simulink model "LQR"  (R2023a)
settings: Solver=ode23t  StartTime=0.0  StopTime=1.1  MaxStep=0.1  RelTol=1e-4
undefined symbols (not defined in the file): LQR_parameters, State_space
settings Model: Creator=ПК  LastModifiedBy=ПК

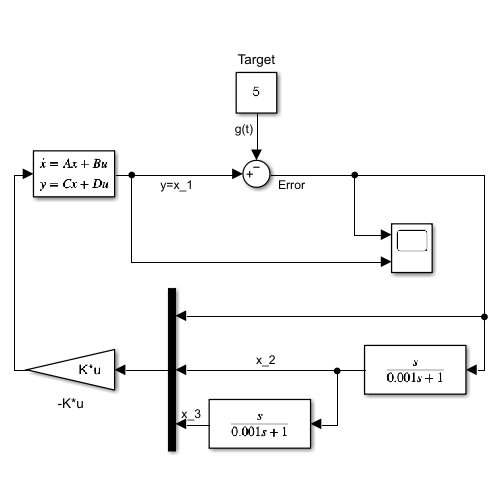
[thumbnail: Simulink's stored preview of the top-level diagram]
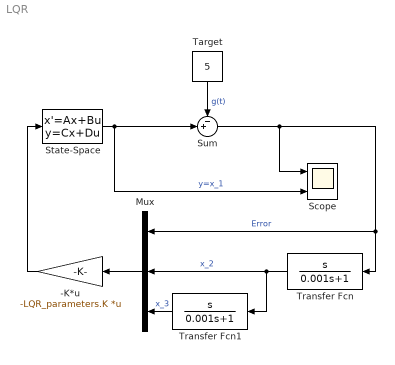
== system LQR ==
  -K*u : Gain  Gain=-LQR_parameters.K  Multiplication=Matrix(K*u)
  Mux : Mux  Inputs=3
  Scope : Scope  NumInputPorts=2
  State-Space : StateSpace  A=State_space.A  B=State_space.B  C=State_space.C  D=State_space.D  InitialCondition=0
  Sum : Sum  Inputs=-+|
  Target : Constant  Value=5
  Transfer Fcn : TransferFcn  Numerator=[1 0]  Denominator=[0.001 1]
  Transfer Fcn1 : TransferFcn  Numerator=[1 0]  Denominator=[0.001 1]
  wires:
  Mux/1 -> -K*u/1
  Transfer Fcn/1 -> Transfer Fcn1/1, Mux/2  "x_2"
  Target/1 -> Sum/1  "g(t)"
  -K*u/1 -> State-Space/1
  State-Space/1 -> Sum/2, Scope/2  "y=x_1"
  Sum/1 -> Scope/1, Transfer Fcn/1, Mux/1  "Error"
  Transfer Fcn1/1 -> Mux/3  "x_3"
